simulink model "s0502_rollest_vertacc"  (R2021a)
settings: Solver=FixedStepAuto  StartTime=0.0  StopTime=10.0  FixedStep=0.001  RelTol=1e-3
undefined symbols (not defined in the file or in its folder): g
libraries: CarMaker4SL x33, dspfdesign x1
settings Model: Creator=jason  LastModifiedBy=jason

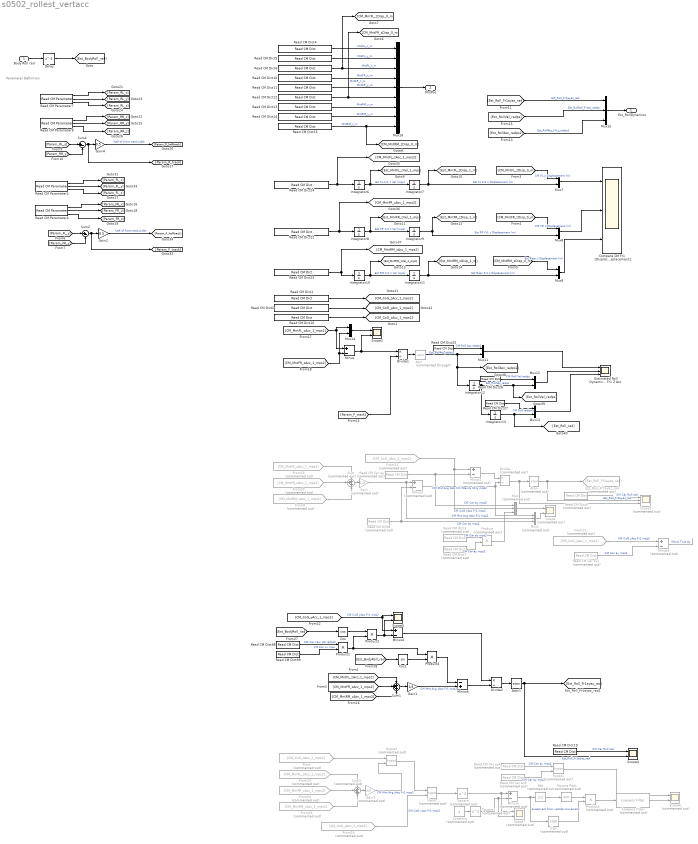
== system s0502_rollest_vertacc ==
  note: Parameter Definition
  Body Roll rad : Inport
  Abs : Abs  Commented=on
  Asin : Trigonometry  Commented=through  Operator=asin
  Atan : Trigonometry  Commented=on  Operator=atan
  Atan1 : Trigonometry  Operator=atan
  Compare CM Fr1 zDisplacement and Estimated Displacement1 : Scope  NumInputPorts=3
  Constant : Constant  Commented=on  Value=g
  Cos : Trigonometry  Operator=cos
  Cos1 : Trigonometry
  Delay : Delay  DelayLength=1
  Divide : Product  Commented=on  Inputs=*/
  Divide1 : Product  Inputs=*/
  Divide2 : Product  Inputs=*/
  Est_Roll_Fr1ayaz_rad : Goto  Commented=on  GotoTag=Est_Roll_Fr1ayaz_rad
  Estimated Roll Dynamics from Fr1 Z Acc : Scope  NumInputPorts=3
  From : From  Commented=on  GotoTag=CM_CoG_xAcc_1_mps2
  From12 : From  Commented=on  GotoTag=CM_CoG_yAcc_1_mps2
  From19 : From  Commented=on  GotoTag=CM_MntFL_zAcc_1_mps2
  From20 : From  Commented=on  GotoTag=CM_MntFR_zAcc_1_mps2
  From21 : From  Commented=on  GotoTag=CM_CoG_yAcc_1_mps2
  From23 : From  Commented=on  GotoTag=CM_MntFL_zAcc_1_mps2
  From24 : From  Commented=on  GotoTag=CM_MntFR_zAcc_1_mps2
  From25 : From  Commented=on  GotoTag=CM_MntRM_zAcc_1_mps2
  From26 : From  Commented=on  GotoTag=CM_CoG_yAcc_1_mps2
  From8 : From  Commented=on  GotoTag=CM_MntRM_zAcc_1_mps2
  Gain : Gain  Commented=on  Gain=1/3
  Gain1 : Gain  Gain=1/3
  Gain2 : Gain  Gain=0.5
  Gain3 : Gain  Commented=on  Gain=1/3
  Gain4 : Gain  Gain=0.5
  Hypot : Math  Commented=on  Operator=hypot  SaturateOnIntegerOverflow=on
  Hypot1 : Math  Commented=on  Operator=hypot  SaturateOnIntegerOverflow=on
  Hypot2 : Math  Commented=on  Operator=hypot  SaturateOnIntegerOverflow=on
  Integrator{6..13} (8 alike) : Integrator
  Lowpass Filter : dspfdesign/Lowpass Filter  Commented=on  FilterType=FIR  DesignForMinimumOrder=on  FilterOrder=50  PassbandFrequency=8e3  StopbandFrequency=12e3  PassbandRipple=0.1  StopbandAttenuation=80  InheritSampleRate=off  SampleRate=44100  SimulateUsing=Interpreted execution  roundingMode=Floor  coeffsDataTypeStr=fixdt(1,16)
  Minus : Sum  Inputs=+-
  Minus{1..3,5} (4 alike) : Sum  Commented=on  Inputs=+-
  Minus4 : Sum  Inputs=+-
  Minus6 : Sum  Inputs=-+
  Mux : Mux  Commented=on  Inputs=3
  Mux1 : Mux  Commented=on  Inputs=3
  Mux{7..9,11..14} (7 alike) : Mux  Inputs=2
  Mux15 : Mux  Inputs=3
  Mux16 : Mux  Inputs=9
  Product : Product  Commented=on
  Product1 : Product
  Product2 : Product
  Product3 : Product  Commented=on
  Product4 : Product
  Read CM Car ay : CarMaker4SL/Read CM Dict  Commented=on  xname=Car.ay  xsync=off  xstime=Continuous
  Read CM Car ay1 : CarMaker4SL/Read CM Dict  Commented=on  xname=Car.ay  xsync=off  xstime=Continuous
  Read CM Car ay4 : CarMaker4SL/Read CM Dict  Commented=on  xname=Car.ay  xsync=off  xstime=Continuous
  Read CM Car ay5 : CarMaker4SL/Read CM Dict  Commented=on  xname=Car.az  xsync=off  xstime=Continuous
  Read CM Dict1 : CarMaker4SL/Read CM Dict  xname=Sensor.Inertial.IN_CoG.Acc_B.z  xsync=off  xstime=Continuous
  Read CM Dict10 : CarMaker4SL/Read CM Dict  xname=Sensor.Inertial.IN_MntFR.Pos_0.x  xsync=off  xstime=Continuous
  Read CM Dict11 : CarMaker4SL/Read CM Dict  xname=Sensor.Inertial.IN_MntFR.Pos_0.y  xsync=off  xstime=Continuous
  Read CM Dict12 : CarMaker4SL/Read CM Dict  xname=Sensor.Inertial.IN_MntFR.Pos_0.z  xsync=off  xstime=Continuous
  Read CM Dict13 : CarMaker4SL/Read CM Dict  xname=Sensor.Inertial.IN_MntRM.Pos_0.x  xsync=off  xstime=Continuous
  Read CM Dict14 : CarMaker4SL/Read CM Dict  xname=Sensor.Inertial.IN_MntRM.Pos_0.y  xsync=off  xstime=Continuous
  Read CM Dict15 : CarMaker4SL/Read CM Dict  xname=Sensor.Inertial.IN_MntRM.Pos_0.z  xsync=off  xstime=Continuous
  Read CM Dict16 : CarMaker4SL/Read CM Dict  xname=Sensor.Inertial.IN_CoG.Acc_B.x  xsync=off  xstime=Continuous
  Read CM Dict19 : CarMaker4SL/Read CM Dict  xname=Car.Roll  xsync=off  xstime=Continuous
  Read CM Dict2 : CarMaker4SL/Read CM Dict  xname=Sensor.Inertial.IN_CoG.Acc_B.y  xsync=off  xstime=Continuous
  Read CM Dict22 : CarMaker4SL/Read CM Dict  xname=Sensor.Inertial.IN_MntFR.Acc_B.z  xsync=off  xstime=Continuous
  Read CM Dict23 : CarMaker4SL/Read CM Dict  xname=Sensor.Inertial.IN_MntRM.Acc_B.z  xsync=off  xstime=Continuous
  Read CM Dict24 : CarMaker4SL/Read CM Dict  xname=Sensor.Inertial.IN_MntFL.Acc_B.z  xsync=off  xstime=Continuous
  Read CM Dict25 : CarMaker4SL/Read CM Dict  xname=Car.RollAcc  xsync=off  xstime=Continuous
  Read CM Dict26 : CarMaker4SL/Read CM Dict  xname=Car.RollVel  xsync=off  xstime=Continuous
  Read CM Dict27 : CarMaker4SL/Read CM Dict  xname=Car.Roll  xsync=off  xstime=Continuous
  Read CM Dict3 : CarMaker4SL/Read CM Dict  Commented=on  xname=Car.vx  xsync=off  xstime=Continuous
  Read CM Dict4 : CarMaker4SL/Read CM Dict  xname=Sensor.Inertial.IN_MntFL.Pos_0.x  xsync=off  xstime=Continuous
  Read CM Dict5 : CarMaker4SL/Read CM Dict  xname=Sensor.Inertial.IN_MntFL.Pos_0.y  xsync=off  xstime=Continuous
  Read CM Dict6 : CarMaker4SL/Read CM Dict  xname=Sensor.Inertial.IN_MntFL.Pos_0.z  xsync=off  xstime=Continuous
  Read CM Dict7 : CarMaker4SL/Read CM Dict  Commented=on  xname=Car.YawRate  xsync=off  xstime=Continuous
  Read CM Dict8 : CarMaker4SL/Read CM Dict  Commented=on  xname=Car.az  xsync=off  xstime=Continuous
  Read CM Dict9 : CarMaker4SL/Read CM Dict  Commented=on  xname=Car.Roll  xsync=off  xstime=Continuous
  Read CM Dict98 : CarMaker4SL/Read CM Dict  xname=Car.YawVel  xsync=off  xstime=Continuous
  Read CM Dict99 : CarMaker4SL/Read CM Dict  xname=Car.vx  xsync=off  xstime=Continuous
  Read CM Parameter2 : CarMaker4SL/Read CM Parameter  xfile=Vehicle  xkey=WheelCarrier.fl.pos  xnout=3  xdefaults=eps  xmuxed=off  xstime=Continuous
      settings: SourceProductName=CarMaker4SL
  Read CM Parameter4 : CarMaker4SL/Read CM Parameter  xfile=Vehicle  xkey=WheelCarrier.fr.pos  xnout=3  xdefaults=eps  xmuxed=off  xstime=Continuous
      settings: SourceProductName=CarMaker4SL
  Read CM Parameter7 : CarMaker4SL/Read CM Parameter  xfile=Vehicle  xkey=WheelCarrier.rl.pos  xnout=3  xdefaults=eps  xmuxed=off  xstime=Continuous
      settings: SourceProductName=CarMaker4SL
  Read CM Parameter8 : CarMaker4SL/Read CM Parameter  xfile=Vehicle  xkey=WheelCarrier.rr.pos  xnout=3  xdefaults=eps  xmuxed=off  xstime=Continuous
      settings: SourceProductName=CarMaker4SL
  Scope : Scope  Commented=on  NumInputPorts=2
  Scope1 : Scope  Commented=on  NumInputPorts=3
  Scope2 : Scope  NumInputPorts=2
  Scope4 : Scope  NumInputPorts=2
  Scope5 : Scope  NumInputPorts=2
  Scope6 : Scope  Commented=on  NumInputPorts=2
  Scope7 : Scope  Commented=on  NumInputPorts=2
  Sign : Signum  Commented=on
  Square : Math  Commented=on  Operator=square  SaturateOnIntegerOverflow=on
  Square Root : Sqrt  Commented=on  SaturateOnIntegerOverflow=on
  Square1 : Math  Commented=on  Operator=square  SaturateOnIntegerOverflow=on
  Sum : Sum  Commented=on  Inputs=+++
  Sum1 : Sum  Inputs=+++
  Sum2 : Sum  Inputs=|+-
  Sum3 : Sum  Commented=on  Inputs=+++
  Sum4 : Sum  Inputs=|+-
  Est_RollDynamics : Outport
  MntPos : Outport  Port=2
  wires:
  Read CM Dict4/1 -> Mux16/1  "MntFL_x_m"
  Read CM Dict5/1 -> Mux16/2  "MntFL_y_m"
  Read CM Dict6/1 -> Mux16/3, [CM_MntFL_zDisp_0_m]  "MntFL_z_m"
  Read CM Dict11/1 -> Mux16/5  "MntFR_y_m"
  Read CM Dict12/1 -> Mux16/6, [CM_MntFR_zDisp_0_m]  "MntFR_z_m"
  Read CM Dict13/1 -> Mux16/7  "MntRM_x_m"
  Read CM Dict14/1 -> Mux16/8  "MntRM_y_m"
  Read CM Dict15/1 -> Mux16/9, [CM_MntRM_zDisp_0_m]  "MntRM_z_m"
  [CM_MntRM_zDisp_0_m] -> Mux9/1  "Est Rear z Displacement (m)"
  [CM_MntFL_zDisp_0_m] -> Mux7/1  "CM FL z Displacement (m)"
  Mux7/1 -> Compare CM Fr1 zDisplacement and Estimated Displacement1/1
  Mux8/1 -> Compare CM Fr1 zDisplacement and Estimated Displacement1/2
  Mux9/1 -> Compare CM Fr1 zDisplacement and Estimated Displacement1/3
  [CM_MntFR_zDisp_0_m] -> Mux8/1  "CM FR z Displacement (m)"
  Integrator7/1 -> [Est_MntFL_zDisp_1_m], Mux7/2  "Est FL Fr1 z Displacement (m)"
  Integrator8/1 -> [Est_MntFR_zVel_1_mps], Integrator9/1  "Est FR Fr1 z Vel (mps)"
  Integrator11/1 -> Mux9/2, [Est_MntRM_zDisp_1_m]  "Est Rear Fr1 z Displacement (m)"
  Integrator10/1 -> [Est_MntRM_zVel_1_mps], Integrator11/1  "Est RM Fr1 z Vel (mps)"
  Integrator6/1 -> [Est_MntFL_zVel_1_mps], Integrator7/1  "Est FL Fr1 z Vel (mps)"
  Integrator9/1 -> [Est_MntFR_zDisp_1_m], Mux8/2  "Est FR Fr1 z Displacement (m)"
  Sum2/1 -> Gain2/1, [Param_F_track]
  Read CM Parameter4/2 -> [Param_FR_y]
  Sum4/1 -> Gain4/1, [Param_R_track]
  [Param_FL_y] -> Sum2/1
  Read CM Parameter2/1 -> [Param_FL_x]
  Read CM Parameter8/2 -> [Param_RR_y]
  Read CM Parameter7/2 -> [Param_RL_y]
  Read CM Parameter8/3 -> [Param_RR_z]
  Gain2/1 -> [Param_F_halftrack]  "half of front trackwidth"
  Read CM Parameter7/3 -> [Param_RL_z]
  Read CM Parameter4/1 -> [Param_FR_x]
  Read CM Parameter4/3 -> [Param_FR_z]
  Read CM Parameter7/1 -> [Param_RL_x]
  [Param_FR_y] -> Sum2/2
  Gain4/1 -> [Param_R_halftrack]  "half of front trackwidth"
  [Param_RR_y] -> Sum4/2
  Read CM Parameter2/2 -> [Param_FL_y]
  Read CM Parameter2/3 -> [Param_FL_z]
  [Param_RL_y] -> Sum4/1
  Read CM Parameter8/1 -> [Param_RR_x]
  Read CM Dict23/1 -> [CM_MntRM_zAcc_1_mps2], Integrator10/1
  Read CM Dict24/1 -> [CM_MntFL_zAcc_1_mps2], Integrator6/1
  Read CM Dict22/1 -> [CM_MntFR_zAcc_1_mps2], Integrator8/1
  [CM_MntFL_zAcc_1_mps2] -> Mux14/1, Minus/1
  [CM_MntFR_zAcc_1_mps2] -> Mux14/2, Minus/2
  [Param_F_track] -> Divide1/2
  Divide1/1 -> Asin/1
  Asin/1 -> Mux11/2, [Est_RollAcc_radps2], Integrator12/1  "Est_RollAcc_radps2"
  Read CM Dict25/1 -> Mux11/1  "CM Roll Acc radps2"
  Mux11/1 -> Estimated Roll Dynamics from Fr1 Z Acc/1
  Integrator12/1 -> Integrator13/1, [Est_RollVel_radps], Mux12/2  "Est_RollVel_radps"
  Read CM Dict26/1 -> Mux12/1  "CM Roll Vel radps"
  Integrator13/1 -> [Est_Roll_rad], Mux13/2
  Read CM Dict27/1 -> Mux13/1  "CM Roll radians"
  Mux12/1 -> Estimated Roll Dynamics from Fr1 Z Acc/2
  Mux13/1 -> Estimated Roll Dynamics from Fr1 Z Acc/3
  Mux14/1 -> Scope2/1
  Mux15/1 -> Est_RollDynamics/1
  Read CM Dict10/1 -> Mux16/4  "MntFR_x_m"
  Mux16/1 -> MntPos/1
  [Est_Roll_Fr1ayaz_rad] -> Mux15/1  "Est_Roll_Fr1ayaz_rad"
  [Est_RollVel_radps] -> Mux15/2  "Est_RollVel_Fr1az_radps"
  [Est_RollAcc_radps2] -> Mux15/3  "Est_RollAcc_Fr1z_radps2"
  Sum/1 -> Gain/1
  From19/1 -> Sum/1
  From20/1 -> Sum/2
  From8/1 -> Sum/3
  Divide/1 -> Scope1/3, Atan/1
  Atan/1 -> Scope1/2, Est_Roll_Fr1ayaz_rad/1  "Est_Roll_Fr1ayaz_rad"
  Minus2/1 -> Mux1/1, Divide/2  "CM Mnt Avg zAcc Fr1 Gravity Only mps2"
  Read CM Dict1/1 -> [CM_CoG_zAcc_1_mps2]
  From21/1 -> Mux/2, Minus1/1  "CM CoG yAcc Fr1 mps2"
  Read CM Dict2/1 -> [CM_CoG_yAcc_1_mps2]
  Read CM Car ay/1 -> Mux/1, Minus1/2  "CM Car ay mps2"
  Minus1/1 -> Divide/1
  Read CM Dict3/1 -> Product/1  "CM Car ay mps2"
  Read CM Dict7/1 -> Product/2  "CM Car ay mps2"
  Product/1 -> Mux/3
  Mux/1 -> Scope/1
  Gain/1 -> Mux1/2, Minus2/1  "CM Mnt Avg zAcc Fr1 mps2"
  Read CM Dict8/1 -> Minus2/2, Mux1/3  "CM Car az mps2"
  Mux1/1 -> Scope/2
  Minus/1 -> Scope2/2, Divide1/1
  Read CM Dict9/1 -> Scope1/1  "CM Car Roll rad"
  [CM_MntFR_zAcc_1_mps2] -> Sum1/2
  Sum1/1 -> Gain1/1
  From12/1 -> Minus3/1  "CM CoG yAcc Fr1 mps2"
  Gain1/1 -> Minus6/2  "CM Mnt Avg zAcc Fr1 mps2"
  Atan1/1 -> [Est_Roll_Fr1ayaz_rad], Scope4/2  "Est_Roll_Fr1ayaz_rad"
  Read CM Dict19/1 -> Scope4/1  "CM Car Roll rad"
  Divide2/1 -> Atan1/1
  [CM_MntFL_zAcc_1_mps2] -> Sum1/1
  [CM_MntRM_zAcc_1_mps2] -> Sum1/3
  Read CM Car ay1/1 -> Minus3/2  "CM Car ay mps2"
  Minus3/1 -> ?  "Minus True Ay"
  Read CM Dict98/1 -> Product1/1  "CM Car Yaw Vel radps2"
  [CM_CoG_yAcc_1_mps2] -> Scope5/1, Minus4/1  "CM CoG yAcc Fr1 mps2"
  Read CM Dict99/1 -> Product1/2  "CM Car vx mps"
  Product1/1 -> Product2/2, Product4/1
  Minus4/1 -> Divide2/1
  Cos/1 -> Product2/1
  Product2/1 -> Minus4/2, Scope5/2
  Gain3/1 -> Hypot2/2  "CM Mnt Avg zAcc Fr1 mps2"
  From24/1 -> Sum3/2
  Sum3/1 -> Gain3/1
  From25/1 -> Sum3/3
  From23/1 -> Sum3/1
  From26/1 -> Hypot/2  "CM CoG yAcc Fr1 mps2"
  Hypot/1 -> Square/1
  Constant/1 -> Square1/1
  Minus5/1 -> Sign/1, Abs/1  "excess acc from vehicle movement"
  Read CM Car ay4/1 -> Hypot1/1  "CM Car ay mps2"
  Read CM Car ay5/1 -> Hypot1/2  "CM Car ay mps2"
  Hypot1/1 -> Scope6/1
  Square/1 -> Scope7/1, Minus5/1
  Square1/1 -> Scope7/2, Minus5/2
  Square Root/1 -> Product3/1
  Abs/1 -> Square Root/1
  Sign/1 -> Product3/2
  Product3/1 -> Lowpass Filter/1
  Lowpass Filter/1 -> Scope6/2
  Read CM Dict16/1 -> [CM_CoG_xAcc_1_mps2]
  From/1 -> Hypot2/1
  Hypot2/1 -> Hypot/1
  Delay/1 -> [Est_BodyRoll_rad]
  Body Roll rad/1 -> Delay/1
  [Est_BodyRoll_rad] -> Cos/1
  Minus6/1 -> Divide2/2
  Cos1/1 -> Product4/2
  [Est_BodyRoll_rad] -> Cos1/1
  Product4/1 -> Minus6/1
